simulink model "attempt_at_model"  (R2024a)
settings: Solver=FixedStepAuto  StartTime=0.0  StopTime=inf  RelTol=1e-3
model workspace (MAT data in the model file):
  SL_ROS_VariableLengthArrays_MaxSizes.CommonInfo.ArrayTruncateAction = 'EmitWarning'
  SL_ROS_VariableLengthArrays_MaxSizes.MsgTypeMap = containers.Map
  SL_ROS_VariableLengthArrays_MaxSizes.MsgTypeMap.serialization.keys = {'sensor_msgs/CompressedImage'}
  SL_ROS_VariableLengthArrays_MaxSizes.MsgTypeMap.serialization.values{1}(1).PropertyName = 'data'
  SL_ROS_VariableLengthArrays_MaxSizes.MsgTypeMap.serialization.values{1}(1).DataType = 'uint8'
  SL_ROS_VariableLengthArrays_MaxSizes.MsgTypeMap.serialization.values{1}(1).MaxLength = 87917
  SL_ROS_VariableLengthArrays_MaxSizes.MsgTypeMap.serialization.values{1}(2).PropertyName = 'format'
  SL_ROS_VariableLengthArrays_MaxSizes.MsgTypeMap.serialization.values{1}(2).DataType = 'uint8'
  SL_ROS_VariableLengthArrays_MaxSizes.MsgTypeMap.serialization.values{1}(2).MaxLength = 128
  SL_ROS_VariableLengthArrays_MaxSizes.MsgTypeMap.serialization.uniformity = 0
  SL_ROS_VariableLengthArrays_MaxSizes.MsgTypeMap.serialization.keyType = 'char'
  SL_ROS_VariableLengthArrays_MaxSizes.MsgTypeMap.serialization.valueType = 'any'
undefined symbols (not defined in the file): angular, fractalcoef, linear, theta, x, y
libraries: ros2lib x19, instrumentlib x5, mspsensorlib x1, visionsinks x1
settings Model: Creator=RedBlueBerry177  LastModifiedBy=ejsui
settings OptimizationCC: EnhancedBackFolding=on  PassReuseOutputArgsAs=Individual arguments  ZeroExternalMemoryAtStartup=off  ZeroInternalMemoryAtStartup=off  MaxStackSize=64  OptimizeBlockOrder=speed  DifferentSizesBufferReuse=on  OptimizationCustomize=off  EfficientTunableParamExpr=on
settings DebuggingCC: ParameterTunabilityLossMsg=error
settings SFSimCC: MATLABDynamicMemAlloc=off  SimTargetLang=C++
settings RTWCC: Description=Embedded Coder  SystemTargetFile=ert.tlc  HardwareBoard=Robot Operating System 2 (ROS 2)  TLCOptions="-aInlineSetEventsForThisBaseRateFcn=TLC_FALSE -aSuppressMultiTaskScheduler=TLC_FALSE  -aRateBasedStepFcn=0"  TemplateMakefile=ert_default_tmf  Toolchain=Colcon Tools  TargetLang=C++  GPUComputeCapability=3.5
settings CodeAppCC: ForceParamTrailComments=on  IgnoreCustomStorageClasses=off  OperatorAnnotations=on  SimulinkDataObjDesc=on  SFDataObjDesc=on  InsertBlockDesc=on
settings ERTTargetCC: CodeInterfacePackaging=C++ class  RootIOFormat=Structure reference

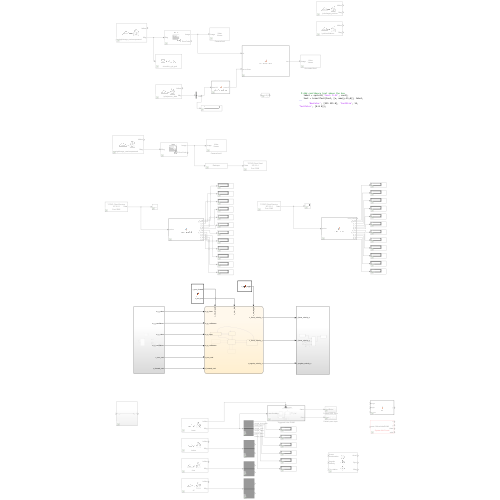
[thumbnail: Simulink's stored preview of the top-level diagram]
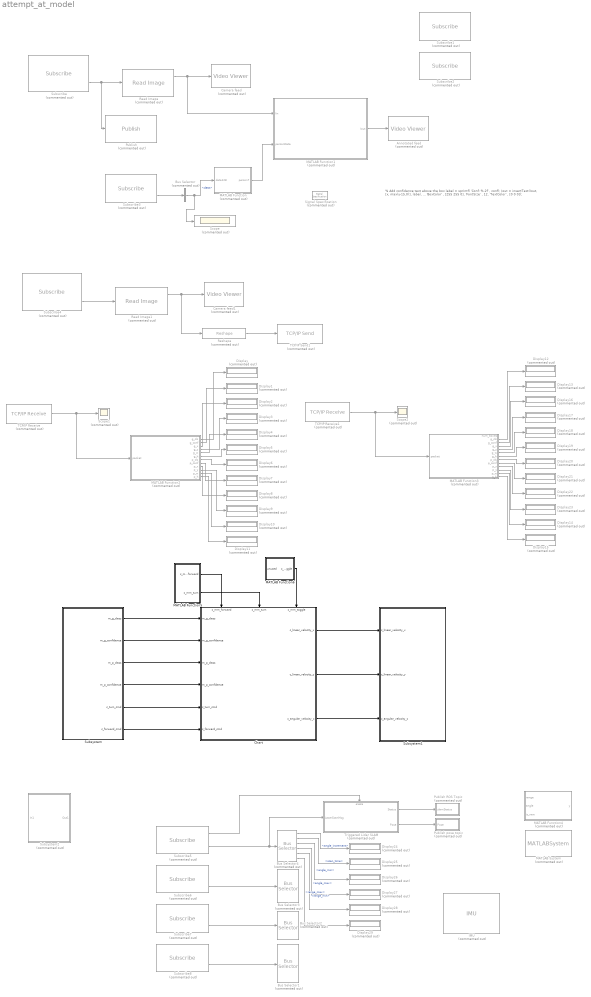
== system attempt_at_model ==
  note: % Add confidence text above the box
      | label = sprintf( 'Conf: %.2f' , conf);
      | Iout = insertText(Iout, [x, max(y-15,0)], label, ...
      | 'BoxColor' , [255 255 0], 'FontSize' , 12, 'TextColor' , [0 0 0]);
  Annotated feed : VideoViewer  Commented=on  FigPos=[1005 760 624 399]
  Bus Selector : BusSelector  Commented=on  OutputSignals=data
  Bus Selector1 : BusSelector  Commented=on  OutputSignals=signal1,signal2
  Bus Selector2 : BusSelector  Commented=on  OutputSignals=signal1,signal2
  Bus Selector3 : BusSelector  Commented=on  OutputSignals=signal1,signal2
  Bus Selector4 : BusSelector  Commented=on  OutputSignals=angle_increment,scan_time,angle_min,angle_max,range_min,range_max
  Camera feed : VideoViewer  Commented=on  FigPos=[409 769 608 539]
  Camera feed1 : VideoViewer  Commented=on  FigPos=[409 769 608 539]
  Chart : Stateflow chart  TreatAsAtomicUnit=on
      settings: PortSchema="{\"entries\":[{\"content\":{\"sides\":[{\"content\":{\"connectorIds\":[\"In4\",\"In5\",\"In6\",\"In7\",\"In8\",\"In9\"]},\"type\":\"ConnectorPlacement.EquallySpacedRectSide\",\"uuid\":\"6869af31-0483-4a0d-a5aa-348304382b03\"},{\"content\":{\"connectorIds\":[\"Out1\",\"Out2\",\"Out3\"],\"side\":\"RIGHT\"},\"type\":\"ConnectorPlacement.EquallySpacedRectSide\",\"uuid\":\"19448461-0885-46d3-901b-79cbd3d2f2eb\"},{\"content\":{\"connectorIds\":[\"In1\",\"In2\",\"In3\"],\"side\":\"TOP\"},\"type\":\"ConnectorPlacement.EquallySpacedRectSide\",\"uuid\":\"dcdfc426-3300-4bb7-b0c9-b15241839ab0\"}]},\"type\":\"ConnectorPlacement.EquallySpacedConnector\",\"uuid\":\"e0f68e20-794f-48c9-96e4-1765267eb054\"}],\"packageUris\":[\"http://schema.mathworks.com/mf0/Connector/R2020b\"],\"version\":\"1.0\"}"
  Display{,1..29} (30 alike) : Display  Commented=on
  IMU : mspsensorlib/IMU  Commented=on  DispRefFrame=NED  TemperaturePort=off  Temperature=25  MagneticFieldPort=off  MagneticFieldNED=[ 27.5550, -2.4169, -16.0849 ]  MagneticFieldENU=[ -2.4169, 27.5550, 16.0849 ]  SeedDouble=67  SimulateUsing=Interpreted execution  AccelParamsMeasurementRange=Inf  AccelParamsResolution=0  AccelParamsConstantBias=[ 0, 0, 0 ]  AccelParamsAxesMisalignment=[ 100, 0, 0; 0, 100, 0; 0, 0, 100 ]  AccelParamsNoiseDensity=[ 0, 0, 0 ]  AccelParamsBiasInstability=[ 0, 0, 0 ]  AccelParamsBiasInstabilityNumerator=fractalcoef().Numerator  AccelParamsBiasInstabilityDenominator=fractalcoef().Denominator  AccelParamsRandomWalk=[ 0, 0, 0 ]  AccelParamsNoiseType=double-sided  AccelParamsTemperatureBias=[ 0, 0, 0 ]  AccelParamsTemperatureScaleFactor=[ 0, 0, 0 ]  GyroParamsMeasurementRange=Inf  GyroParamsResolution=0  GyroParamsConstantBias=[ 0, 0, 0 ]  GyroParamsAxesMisalignment=[ 100, 0, 0; 0, 100, 0; 0, 0, 100 ]  GyroParamsAccelerationBias=[ 0, 0, 0 ]  GyroParamsNoiseDensity=[ 0, 0, 0 ]  GyroParamsBiasInstability=[ 0, 0, 0 ]  GyroParamsBiasInstabilityNumerator=fractalcoef().Numerator  GyroParamsBiasInstabilityDenominator=fractalcoef().Denominator  GyroParamsRandomWalk=[ 0, 0, 0 ]  GyroParamsNoiseType=double-sided  GyroParamsTemperatureBias=[ 0, 0, 0 ]  GyroParamsTemperatureScaleFactor=[ 0, 0, 0 ]  MagParamsMeasurementRange=Inf  MagParamsResolution=0  MagParamsConstantBias=[ 0, 0, 0 ]  MagParamsAxesMisalignment=[ 100, 0, 0; 0, 100, 0; 0, 0, 100 ]  MagParamsNoiseDensity=[ 0, 0, 0 ]  MagParamsBiasInstability=[ 0, 0, 0 ]  MagParamsBiasInstabilityNumerator=fractalcoef().Numerator  MagParamsBiasInstabilityDenominator=fractalcoef().Denominator  MagParamsRandomWalk=[ 0, 0, 0 ]  MagParamsNoiseType=double-sided  MagParamsTemperatureBias=[ 0, 0, 0 ]  MagParamsTemperatureScaleFactor=[ 0, 0, 0 ]
  MATLAB Function : MATLAB Function  Commented=on  TreatAsAtomicUnit=on
  MATLAB Function1 : MATLAB Function  Commented=on  TreatAsAtomicUnit=on
  MATLAB Function2 : MATLAB Function  Commented=on  TreatAsAtomicUnit=on
  MATLAB Function3 : MATLAB Function  Commented=on  TreatAsAtomicUnit=on
  MATLAB Function4 : MATLAB Function  Commented=on  TreatAsAtomicUnit=on
  MATLAB Function5 : MATLAB Function  TreatAsAtomicUnit=on
  MATLAB Function6 : MATLAB Function  TreatAsAtomicUnit=on
  MATLAB System : MATLABSystem  Commented=on  System=OnlineLidarSLAM  MapResolution=10  MaxRange=8.0  SimulateUsing=Code generation
      mask Type: OnlineLidarSLAM
      mask Display:
      | disp('OnlineLidarSLAM');
      | port_label('input',1,'scan');
      | port_label('output',1,'x');
      | port_label('output',2,'y');
      | port_label('output',3,'theta');
      | port_label('output',4,'valid');
  Publish : ros2lib/Publish  Commented=on  topicSource=Specify your own  topic=/simulink_rgb_pub  messageType=sensor_msgs/CompressedImage  QOSHistory=Keep last  QOSDepth=1  QOSReliability=Reliable  QOSDurability=Volatile  QOSDeadline=Inf  QOSLifespan=Inf  QOSLiveliness=Automatic  QOSLeaseDuration=Inf  QOSAvoidROSNamespaceConventions=off
  Publish ROS Topic : Subsystem  Commented=on
  Publish pose topic : Subsystem  Commented=on
  Read Image : ros2lib/Read Image  Commented=on  MaximumImageSize=[480,640]  ImageEncoding=rgb8  ShowAlphaOutput=off  ShowErrorCodeOutput=on  VariableSizeOutputs=off
  Read Image1 : ros2lib/Read Image  Commented=on  MaximumImageSize=[480,640]  ImageEncoding=rgb8  ShowAlphaOutput=off  ShowErrorCodeOutput=on  VariableSizeOutputs=off
  Reshape : Reshape  Commented=on  OutputDimensionality=Customize  OutputDimensions=[480 640 3]
  Scope : Scope  Commented=on
  Scope1 : Scope  Commented=on
  Scope2 : Scope  Commented=on
  Signal Specification : SignalSpecification  Commented=on  OutDataTypeStr=single  Dimensions=[1 7]
  Subscribe : ros2lib/Subscribe  Commented=on  topicSource=Select from ROS network  topic=/depth_cam/rgb/image_raw/compressed  messageType=sensor_msgs/CompressedImage  sampleTime=-1  QOSHistory=Keep last  QOSDepth=1  QOSReliability=Best effort  QOSDurability=Volatile  QOSDeadline=Inf  QOSLifespan=Inf  QOSLiveliness=Automatic  QOSLeaseDuration=Inf  QOSAvoidROSNamespaceConventions=off
  Subscribe1 : ros2lib/Subscribe  Commented=on  topicSource=Select from ROS network  topic=/yolo/target_position  messageType=geometry_msgs/Point  sampleTime=-1  QOSHistory=Keep last  QOSDepth=1  QOSReliability=Reliable  QOSDurability=Volatile  QOSDeadline=Inf  QOSLifespan=Inf  QOSLiveliness=Automatic  QOSLeaseDuration=Inf  QOSAvoidROSNamespaceConventions=off
  Subscribe2 : ros2lib/Subscribe  Commented=on  topicSource=Select from ROS network  topic=/yolo/confidence  messageType=std_msgs/Float32  sampleTime=-1  QOSHistory=Keep last  QOSDepth=1  QOSReliability=Reliable  QOSDurability=Volatile  QOSDeadline=Inf  QOSLifespan=Inf  QOSLiveliness=Automatic  QOSLeaseDuration=Inf  QOSAvoidROSNamespaceConventions=off
  Subscribe3 : ros2lib/Subscribe  Commented=on  topicSource=Select from ROS network  topic=/yolo/person_data  messageType=std_msgs/Float32MultiArray  sampleTime=-1  QOSHistory=Keep last  QOSDepth=1  QOSReliability=Reliable  QOSDurability=Volatile  QOSDeadline=Inf  QOSLifespan=Inf  QOSLiveliness=Automatic  QOSLeaseDuration=Inf  QOSAvoidROSNamespaceConventions=off
  Subscribe4 : ros2lib/Subscribe  Commented=on  topicSource=Select from ROS network  topic=/depth_cam/rgb/image_raw/compressed  messageType=sensor_msgs/CompressedImage  sampleTime=-1  QOSHistory=Keep last  QOSDepth=1  QOSReliability=Best effort  QOSDurability=Volatile  QOSDeadline=Inf  QOSLifespan=Inf  QOSLiveliness=Automatic  QOSLeaseDuration=Inf  QOSAvoidROSNamespaceConventions=off
  Subscribe5 : ros2lib/Subscribe  Commented=on  topicSource=Select from ROS network  topic=/scan  messageType=sensor_msgs/LaserScan  sampleTime=-1  QOSHistory=Keep last  QOSDepth=1  QOSReliability=Reliable  QOSDurability=Volatile  QOSDeadline=Inf  QOSLifespan=Inf  QOSLiveliness=Automatic  QOSLeaseDuration=Inf  QOSAvoidROSNamespaceConventions=off
  Subscribe6 : ros2lib/Subscribe  Commented=on  topicSource=Select from ROS network  topic=/odom  messageType=nav_msgs/Odometry  sampleTime=-1  QOSHistory=Keep last  QOSDepth=1  QOSReliability=Reliable  QOSDurability=Volatile  QOSDeadline=Inf  QOSLifespan=Inf  QOSLiveliness=Automatic  QOSLeaseDuration=Inf  QOSAvoidROSNamespaceConventions=off
  Subscribe7 : ros2lib/Subscribe  Commented=on  topicSource=Select from ROS network  topic=/imu  messageType=sensor_msgs/Imu  sampleTime=-1  QOSHistory=Keep last  QOSDepth=1  QOSReliability=Reliable  QOSDurability=Volatile  QOSDeadline=Inf  QOSLifespan=Inf  QOSLiveliness=Automatic  QOSLeaseDuration=Inf  QOSAvoidROSNamespaceConventions=off
  Subscribe8 : ros2lib/Subscribe  Commented=on  topicSource=Select from ROS network  topic=/tf  messageType=tf2_msgs/TFMessage  sampleTime=-1  QOSHistory=Keep last  QOSDepth=1  QOSReliability=Reliable  QOSDurability=Volatile  QOSDeadline=Inf  QOSLifespan=Inf  QOSLiveliness=Automatic  QOSLeaseDuration=Inf  QOSAvoidROSNamespaceConventions=off
  Subsystem : Subsystem
  Subsystem1 : Subsystem
  Subsystem2 : Subsystem  Commented=on
  TCP/IP Receive : instrumentlib/TCP//IP Receive  Commented=on  Host=127.0.0.1  Port=5005  DataSize=[56, 1]  DataType=uint8  ASCIIFormatting=%f  Terminator=LF  CustomTerminator=10  ByteOrder=big-endian  EnableBlockingMode=on  Timeout=1000  SampleTime=0.01  SimulateUsing=Interpreted execution
  TCP/IP Receive1 : instrumentlib/TCP//IP Receive  Commented=on  Host=127.0.0.1  Port=5005  DataSize=[52, 1]  DataType=uint8  ASCIIFormatting=%f  Terminator=LF  CustomTerminator=10  ByteOrder=big-endian  EnableBlockingMode=on  Timeout=1000  SampleTime=0.01  SimulateUsing=Interpreted execution
  TCP/IP Send1 : instrumentlib/TCP//IP Send  Commented=on  Host=127.0.0.1  Port=5005  ByteOrder=big-endian  EnableBlockingMode=on  Timeout=10  TransferDelay=off  SimulateUsing=Interpreted execution
  Triggered Lidar SLAM : Subsystem  Commented=on
  wires:
  Subscribe/2 -> Publish/1, Read Image/1
  Read Image/1 -> MATLAB Function1/1(Iin), Camera feed/1
  MATLAB Function1/1(Iout) -> Annotated feed/1
  Subscribe3/2 -> Bus Selector/1
  Bus Selector/1 -> Scope/1, MATLAB Function/1(data128)  "<data>"
  MATLAB Function/1(person7) -> MATLAB Function1/2(personData)
  Subscribe4/2 -> Read Image1/1
  Read Image1/1 -> Reshape/1, Camera feed1/1
  Reshape/1 -> TCP/IP Send1/1
  TCP/IP Receive/1 -> MATLAB Function2/1(packet), Scope1/1
  MATLAB Function2/1(g_cls) -> Display/1
  MATLAB Function2/2(g_conf) -> Display1/1
  MATLAB Function2/3(g_x) -> Display2/1
  MATLAB Function2/4(g_y) -> Display3/1
  MATLAB Function2/5(g_w) -> Display4/1
  MATLAB Function2/6(g_h) -> Display5/1
  MATLAB Function2/7(p_cls) -> Display6/1
  MATLAB Function2/8(p_conf) -> Display7/1
  MATLAB Function2/9(p_x) -> Display8/1
  MATLAB Function2/10(p_y) -> Display9/1
  MATLAB Function2/11(p_w) -> Display10/1
  MATLAB Function2/12(p_h) -> Display11/1
  MATLAB Function3/8(p_cls) -> Display20/1
  MATLAB Function3/12(p_w) -> Display14/1
  MATLAB Function3/11(p_y) -> Display23/1
  MATLAB Function3/9(p_conf) -> Display21/1
  MATLAB Function3/10(p_x) -> Display22/1
  MATLAB Function3/2(g_cls) -> Display12/1
  MATLAB Function3/13(p_h) -> Display15/1
  MATLAB Function3/6(g_w) -> Display18/1
  MATLAB Function3/4(g_x) -> Display16/1
  MATLAB Function3/5(g_y) -> Display17/1
  TCP/IP Receive1/1 -> MATLAB Function3/1(packet), Scope2/1
  MATLAB Function3/3(g_conf) -> Display13/1
  MATLAB Function3/7(g_h) -> Display19/1
  Subsystem/1(m_g_class) -> Chart/4(m_g_class)
  Subsystem/2(m_g_confidence) -> Chart/5(m_g_confidence)
  Subsystem/3(m_p_class) -> Chart/6(m_p_class)
  Subsystem/4(m_p_confidence) -> Chart/7(m_p_confidence)
  Chart/1(c_linear_velocity_x) -> Subsystem1/1(c_linear_velocity_x)
  Chart/2(c_linear_velocity_y) -> Subsystem1/2(c_linear_velocity_y)
  Subsystem/5(c_turn_cmd) -> Chart/8(c_turn_cmd)
  Subsystem/6(c_forward_cmd) -> Chart/9(c_forward_cmd)
  Chart/3(c_angular_velocity_z) -> Subsystem1/3(c_angular_velocity_z)
  Subscribe8/2 -> Bus Selector1/1
  Subscribe7/2 -> Bus Selector2/1
  Subscribe6/2 -> Bus Selector3/1
  Subscribe5/2 -> Triggered Lidar SLAM/1(LaserScanMsg), Bus Selector4/1
  Subscribe5/1 -> Triggered Lidar SLAM/Enable
  Triggered Lidar SLAM/1(Status) -> Publish ROS Topic/1(slamStatus)
  Triggered Lidar SLAM/2(Pose) -> Publish pose topic/1(Pose)
  Bus Selector4/1 -> Display24/1  "<angle_increment>"
  Bus Selector4/2 -> Display25/1  "<scan_time>"
  Bus Selector4/3 -> Display26/1  "<angle_min>"
  Bus Selector4/4 -> Display27/1  "<angle_max>"
  Bus Selector4/5 -> Display28/1  "<range_min>"
  Bus Selector4/6 -> Display29/1  "<range_max>"
  MATLAB Function5/1(c_mm_forward) -> Chart/1(c_mm_forward)
  MATLAB Function5/2(c_mm_turn) -> Chart/2(c_mm_turn)
  MATLAB Function6/1(c_mm_toggle) -> Chart/3(c_mm_toggle)

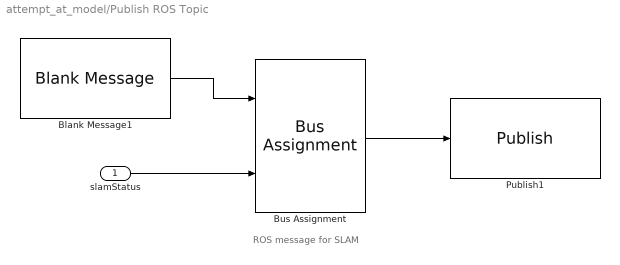
== system attempt_at_model/Publish ROS Topic ==
  note: ROS message for SLAM
  slamStatus : Inport
  Blank Message1 : ros2lib/Blank Message  messageClass=Message  entityType=std_msgs/Int8  messageType=std_msgs/Int8  SampleTime=inf
  Bus Assignment : BusAssignment  AssignedSignals=data
  Publish1 : ros2lib/Publish  topicSource=Specify your own  topic=/slamStatus  messageType=std_msgs/Int8  QOSHistory=Keep last  QOSDepth=1  QOSReliability=Reliable  QOSDurability=Volatile  QOSDeadline=Inf  QOSLifespan=Inf  QOSLiveliness=Automatic  QOSLeaseDuration=Inf  QOSAvoidROSNamespaceConventions=off
  wires:
  slamStatus/1 -> Bus Assignment/2
  Blank Message1/1 -> Bus Assignment/1
  Bus Assignment/1 -> Publish1/1

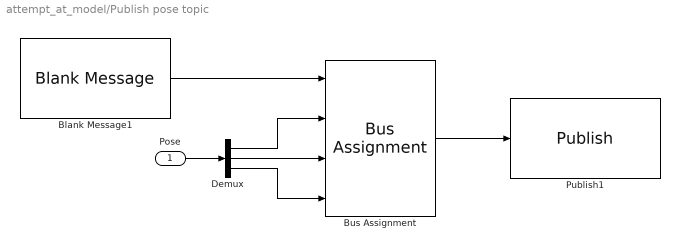
== system attempt_at_model/Publish pose topic ==
  Pose : Inport
  Blank Message1 : ros2lib/Blank Message  messageClass=Message  entityType=geometry_msgs/Pose2D  messageType=geometry_msgs/Pose2D  SampleTime=inf
  Bus Assignment : BusAssignment  AssignedSignals=x,y,theta
  Demux : Demux  Outputs=3
  Publish1 : ros2lib/Publish  topicSource=Specify your own  topic=/pose  messageType=geometry_msgs/Pose2D  QOSHistory=Keep last  QOSDepth=1  QOSReliability=Reliable  QOSDurability=Volatile  QOSDeadline=Inf  QOSLifespan=Inf  QOSLiveliness=Automatic  QOSLeaseDuration=Inf  QOSAvoidROSNamespaceConventions=off
  wires:
  Pose/1 -> Demux/1
  Demux/3 -> Bus Assignment/4
  Demux/1 -> Bus Assignment/2
  Demux/2 -> Bus Assignment/3
  Blank Message1/1 -> Bus Assignment/1
  Bus Assignment/1 -> Publish1/1

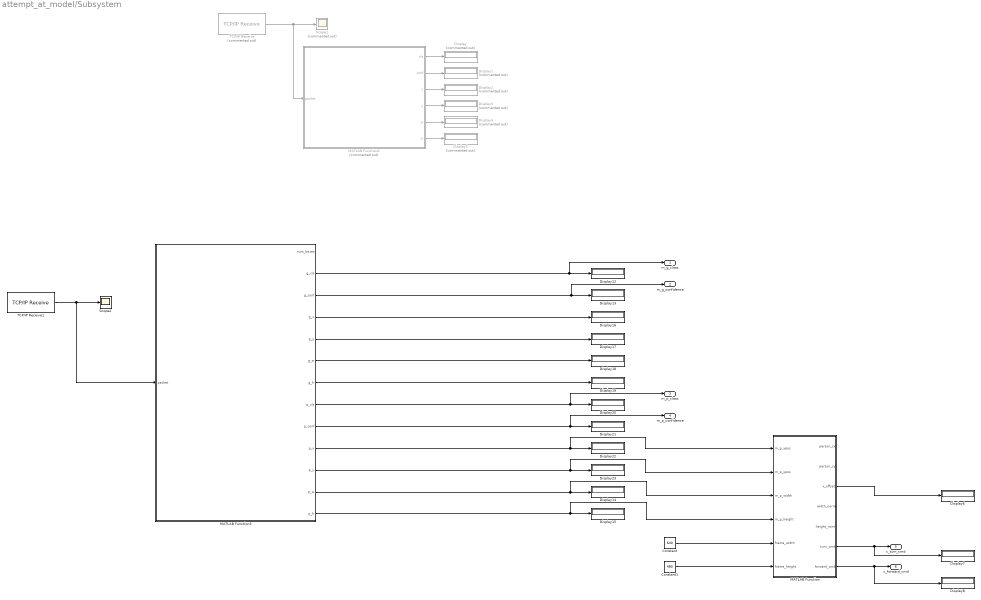
== system attempt_at_model/Subsystem ==
  Constant : Constant  Value=640
  Constant1 : Constant  Value=480
  Display{,1..5} (6 alike) : Display  Commented=on
  Display{6..8,12..23} (15 alike) : Display
  MATLAB Function : MATLAB Function  TreatAsAtomicUnit=on
  MATLAB Function2 : MATLAB Function  Commented=on  TreatAsAtomicUnit=on
  MATLAB Function3 : MATLAB Function  TreatAsAtomicUnit=on
  Scope1 : Scope  Commented=on
  Scope2 : Scope
  TCP/IP Receive : instrumentlib/TCP//IP Receive  Commented=on  Host=127.0.0.1  Port=5005  DataSize=[28, 1]  DataType=uint8  ASCIIFormatting=%f  Terminator=LF  CustomTerminator=10  ByteOrder=big-endian  EnableBlockingMode=on  Timeout=1000  SampleTime=0.01  SimulateUsing=Interpreted execution
  TCP/IP Receive1 : instrumentlib/TCP//IP Receive  Host=127.0.0.1  Port=5005  DataSize=[52, 1]  DataType=uint8  ASCIIFormatting=%f  Terminator=LF  CustomTerminator=10  ByteOrder=big-endian  EnableBlockingMode=on  Timeout=1000  SampleTime=0.01  SimulateUsing=Interpreted execution
  m_g_class : Outport
  m_g_confidence : Outport  Port=2
  m_p_class : Outport  Port=3
  m_p_confidence : Outport  Port=4
  c_turn_cmd : Outport  Port=5
  c_forward_cmd : Outport  Port=6
  wires:
  MATLAB Function2/1(cls) -> Display/1
  MATLAB Function2/4(y) -> Display3/1
  MATLAB Function2/6(h) -> Display5/1
  MATLAB Function2/3(x) -> Display2/1
  MATLAB Function2/5(w) -> Display4/1
  TCP/IP Receive/1 -> MATLAB Function2/1(packet), Scope1/1
  MATLAB Function2/2(conf) -> Display1/1
  MATLAB Function3/9(p_conf) -> m_p_confidence/1, Display21/1
  MATLAB Function3/6(g_w) -> Display18/1
  MATLAB Function3/4(g_x) -> Display16/1
  MATLAB Function3/13(p_h) -> MATLAB Function/4(m_p_height), Display15/1
  MATLAB Function3/10(p_x) -> MATLAB Function/1(m_p_xpos), Display22/1
  MATLAB Function3/7(g_h) -> Display19/1
  MATLAB Function3/8(p_cls) -> m_p_class/1, Display20/1
  MATLAB Function3/11(p_y) -> MATLAB Function/2(m_p_ypos), Display23/1
  MATLAB Function3/3(g_conf) -> m_g_confidence/1, Display13/1
  MATLAB Function3/2(g_cls) -> m_g_class/1, Display12/1
  MATLAB Function3/5(g_y) -> Display17/1
  TCP/IP Receive1/1 -> MATLAB Function3/1(packet), Scope2/1
  MATLAB Function3/12(p_w) -> MATLAB Function/3(m_p_width), Display14/1
  Constant/1 -> MATLAB Function/5(frame_width)
  Constant1/1 -> MATLAB Function/6(frame_height)
  MATLAB Function/3(x_offset) -> Display6/1
  MATLAB Function/6(turn_cmd) -> Display7/1, c_turn_cmd/1
  MATLAB Function/7(forward_cmd) -> Display8/1, c_forward_cmd/1

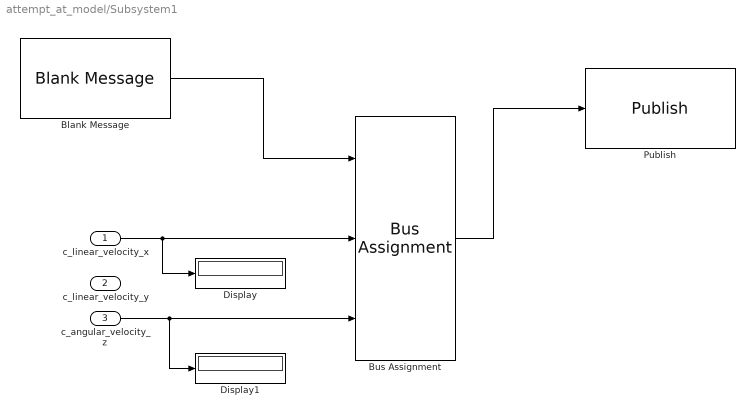
== system attempt_at_model/Subsystem1 ==
  c_linear_velocity_x : Inport
  c_linear_velocity_y : Inport  Port=2
  c_angular_velocity_z : Inport  Port=3
  Blank Message : ros2lib/Blank Message  messageClass=Message  entityType=geometry_msgs/Twist  messageType=geometry_msgs/Twist  SampleTime=inf
  Bus Assignment : BusAssignment  AssignedSignals=linear.x,angular.z
  Display : Display
  Display1 : Display
  Publish : ros2lib/Publish  topicSource=Select from ROS network  topic=/controller/cmd_vel  messageType=geometry_msgs/Twist  QOSHistory=Keep last  QOSDepth=1  QOSReliability=Reliable  QOSDurability=Volatile  QOSDeadline=Inf  QOSLifespan=Inf  QOSLiveliness=Automatic  QOSLeaseDuration=Inf  QOSAvoidROSNamespaceConventions=off
  wires:
  Blank Message/1 -> Bus Assignment/1
  c_linear_velocity_x/1 -> Display/1, Bus Assignment/2
  Bus Assignment/1 -> Publish/1
  c_angular_velocity_z/1 -> Display1/1, Bus Assignment/3

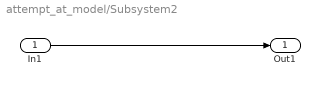
== system attempt_at_model/Subsystem2 ==
  In1 : Inport
  Out1 : Outport
  wires:
  In1/1 -> Out1/1

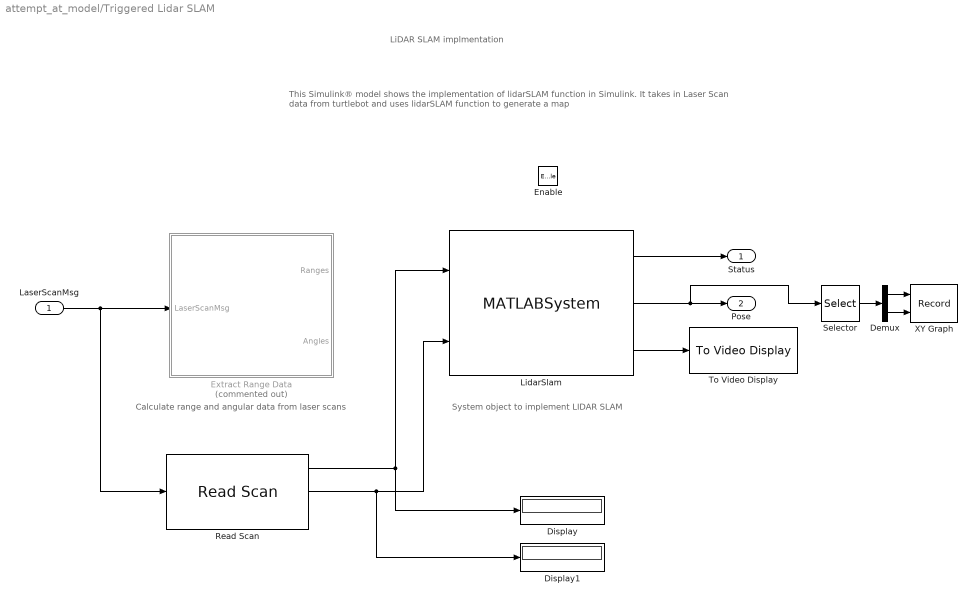
== system attempt_at_model/Triggered Lidar SLAM ==
  note: Calculate range and angular data from laser scans
  note: LiDAR SLAM implmentation
  note: This Simulink® model shows the implementation of lidarSLAM function in Simulink. It takes in Laser Scan data from turtlebot and uses lidarSLAM function to generate a map
  note: System object to implement LIDAR SLAM
  LaserScanMsg : Inport
  Enable : EnablePort  PropagateVarSize=During execution
  Demux : Demux  Outputs=2
  Display : Display
  Display1 : Display
  Extract Range Data : MATLAB Function  Commented=on  TreatAsAtomicUnit=on
  LidarSlam : MATLABSystem  System=LidarSlam_interp  SimulateUsing=Interpreted execution
      mask Type: LidarSlam_interp
      mask Display:
      | disp('LidarSlam_interp');
      | port_label('input',1,'ranges');
      | port_label('input',2,'angles');
      | port_label('output',1,'slamStatus');
      | port_label('output',2,'pose');
      | port_label('output',3,'mapData');
  Read Scan : ros2lib/Read Scan  MaximumArrayLength=1000  ShowAnglesOutput=on  ShowIntensityOutput=off  ShowErrorCodeOutput=on  VariableSizeOutputs=off
  Selector : Selector  InputPortWidth=3  IndexOptions=Index vector (dialog)  Indices=[1 2]  OutputSizes=1
  To Video Display : visionsinks/To Video Display  windowSizeMode=Normal  openAtMdlStart=on  fullScreen=off  videoWindowX=536805376  videoWindowY=536805376  saveWindowSize=off  videoWindowWidth=1000  videoWindowHeight=1000  inputColorFormat=RGB  inputType=Obsolete  imagePorts=One multidimensional signal  OutputDevice=On-screen video monitor  dataOrg=Column-major  isWindowOpen=off
  XY Graph : Record  FileSettingsInternal="{\"entries\":[{\"content\":{\"excelSettings\":{\"content\":{},\"type\":\"Streamout.ExcelSettings\"}},\"type\":\"Streamout.FileSettingStorage\",\"uuid\":\"\"}],\"packageUris\":[\"http:\\/\\/schema.mathworks.com\\/mf0\\/streamout_blocks\\/R2020a\"],\"version\":\"1.0\"}"  Layout=[1 1]  SignalsInternal="{\"entries\":[{\"content\":{\"signals\":[{\"content\":{\"blockPath\":[],\"dimensions\":[1,1],\"domain\":\"\",\"lineColor\":\"#a2142f\",\"plots\":[ 1 ],\"port\":1,\"signalID\":1,\"signalName\":\"Demux:1\"},\"type\":\"RecordBlkView.Signal\",\"uuid\":\"\"},{\"content\":{\"blockPath\":[],\"dimensions\":[1,1],\"domain\":\"\",\"lineColor\":\"#139fff\",\"plots\":[ 1 ],\"port\":2,\"signalID\":2,\"signalName\":\"Demux:2\"},\"type\":\"RecordBlkView.Signal\",\"uuid\":\"\"}]},\"type\":\"RecordBlkView.InputSignals\",\"uuid\":\"\"}],\"packageUris\":[\"http:\\/\\/schema.mathworks.com\\/mf0\\/streamout_blocks\\/R2020a\"],\"version\":\"1.0\"}"  VisualizationBindings="{\"xyplotplugin\":{\"info\":[{\"series\":[{\"bindingParametersList\":[{\"parameter\":\"X-Axis\",\"signalID\":1,\"signalName\":\"Demux:1\"},{\"parameter\":\"Y-Axis\",\"signalID\":2,\"signalName\":\"Demux:2\"}],\"seriesID\":0}],\"subplotID\":1}]}}"  CompatibilityTag=XY  st=-1
  Status : Outport
  Pose : Outport  Port=2
  wires:
  LaserScanMsg/1 -> Read Scan/1, Extract Range Data/1(LaserScanMsg)
  LidarSlam/1 -> Status/1
  LidarSlam/2 -> Pose/1, Selector/1
  Demux/2 -> XY Graph/2
  Demux/1 -> XY Graph/1
  Selector/1 -> Demux/1
  LidarSlam/3 -> To Video Display/1
  Read Scan/1 -> LidarSlam/1, Display/1
  Read Scan/2 -> Display1/1, LidarSlam/2

== stateflow chart attempt_at_model/Chart ==
  state Initial
  state Manual_Mode
    c_linear_velocity_x = c_mm_forward;
    c_angular_velocity_z = c_mm_turn;
  state Path_Planning_and_Navigation [commented out]
  state Idle
    c_linear_velocity_x = 0.0;
    c_linear_velocity_y = 0.0;
    c_angular_velocity_z = 0.0;
  state Follow
    c_linear_velocity_x = c_forward_cmd;
    c_linear_velocity_y = 0;
    c_angular_velocity_z = c_turn_cmd;
  state Mapping_and_Localization [commented out]
  Follow -> Manual_Mode [order 2] : [c_mm_toggle ==1]
  (default) -> Initial
  Initial -> Manual_Mode [order 2] : [c_mm_toggle == 1]
  Manual_Mode -> Initial : [c_mm_toggle == 0]
  Idle -> Manual_Mode [order 2] : [c_mm_toggle == 1]
  Initial -> Idle [order 1] : [(m_g_class == 9) & (m_p_class ==1)]
  Path_Planning_and_Navigation -> Idle [commented out]
  Idle -> Follow [order 1] : [m_g_class == 20]
  Idle -> Path_Planning_and_Navigation [commented out]
  Follow -> Idle [order 1] : [(m_g_class == 13) | (m_p_class == 0)]
  Idle -> Mapping_and_Localization [commented out] : [m_g_class == 13]
  Mapping_and_Localization -> Idle [commented out]
  data: c_mm_forward input; c_mm_turn input; c_mm_toggle input; m_g_class input; m_g_confidence input; m_p_class input; m_p_confidence input; c_linear_velocity_x output; c_linear_velocity_y output; c_turn_cmd input; c_forward_cmd input; c_angular_velocity_z output

== matlab function attempt_at_model/Subsystem/MATLAB Function2 ==
  data: packet input; cls output int32 size=1; conf output single size=1; x output single size=1; y output single size=1; w output single size=1; h output single size=1
function [cls, conf, x, y, w, h] = parse_packet(packet)
    cls  = typecast(packet(5:8), 'int32');       
    conf = typecast(packet(9:12), 'single');
    x    = typecast(packet(13:16), 'single');
    y    = typecast(packet(17:20), 'single');
    w    = typecast(packet(21:24), 'single');
    h    = typecast(packet(25:28), 'single');
end

== matlab function attempt_at_model/MATLAB Function3 ==
  data: num_boxes output uint32 size=1; packet input; g_cls output int32 size=1; g_conf output single size=1; g_x output single size=1; g_y output single size=1; g_w output single size=1; g_h output single size=1; p_cls output int32 size=1; p_conf output single size=1; p_x output single size=1; p_y output single size=1; p_w output single size=1; p_h output single size=1
function [num_boxes, g_cls, g_conf, g_x, g_y, g_w, g_h, p_cls, p_conf, p_x, p_y, p_w, p_h] = parse_packet(packet)

num_boxes = typecast(packet(1:4), 'uint32');

% Person box
p_cls  = typecast(packet(5:8), 'int32');
p_conf = typecast(packet(9:12), 'single');
p_x    = typecast(packet(13:16), 'single');
p_y    = typecast(packet(17:20), 'single');
p_w    = typecast(packet(21:24), 'single');
p_h    = typecast(packet(25:28), 'single');

% Gesture box
g_cls  = typecast(packet(29:32), 'int32');
g_conf = typecast(packet(33:36), 'single');
g_x    = typecast(packet(37:40), 'single');
g_y    = typecast(packet(41:44), 'single');
g_w    = typecast(packet(45:48), 'single');
g_h    = typecast(packet(49:52), 'single');
end

== matlab function attempt_at_model/Subsystem/MATLAB Function3 ==
  data: num_boxes output uint32 size=1; packet input; g_cls output int32 size=1; g_conf output single size=1; g_x output single size=1; g_y output single size=1; g_w output single size=1; g_h output single size=1; p_cls output int32 size=1; p_conf output single size=1; p_x output single size=1; p_y output single size=1; p_w output single size=1; p_h output single size=1
function [num_boxes, g_cls, g_conf, g_x, g_y, g_w, g_h, p_cls, p_conf, p_x, p_y, p_w, p_h] = parse_packet(packet)

num_boxes = typecast(packet(1:4), 'uint32');

% Person box
p_cls  = typecast(packet(5:8), 'int32');
p_conf = typecast(packet(9:12), 'single');
p_x    = typecast(packet(13:16), 'single');
p_y    = typecast(packet(17:20), 'single');
p_w    = typecast(packet(21:24), 'single');
p_h    = typecast(packet(25:28), 'single');

% Gesture box
g_cls  = typecast(packet(29:32), 'int32');
g_conf = typecast(packet(33:36), 'single');
g_x    = typecast(packet(37:40), 'single');
g_y    = typecast(packet(41:44), 'single');
g_w    = typecast(packet(45:48), 'single');
g_h    = typecast(packet(49:52), 'single');
end

== matlab function attempt_at_model/Subsystem/MATLAB Function ==
  data: m_p_xpos input; person_cx output; m_p_ypos input; m_p_width input; m_p_height input; frame_width input; frame_height input; person_cy output; x_offset output; width_norm output; height_norm output; turn_cmd output; forward_cmd output
function [person_cx, person_cy, x_offset, width_norm, height_norm, turn_cmd, forward_cmd] = compute_person_controls(m_p_xpos, m_p_ypos, m_p_width, m_p_height, frame_width, frame_height)
% Computes quantities for following a person in a frame
%
% Inputs:
%   m_p_xpos, m_p_ypos : top-left corner of person bounding box
%   m_p_width, m_p_height : width and height of bounding box
%   frame_width, frame_height : size of camera frame
%
% Outputs:
%   person_cx, person_cy : center of bounding box
%   x_offset : horizontal offset from frame center (pixels)
%   width_norm, height_norm : bounding box size normalized to frame size
%   turn_cmd : command for turning (-1=left, 0=centered, 1=right)
%   forward_cmd : command for forward movement (0=stop, 1=move)

% Compute center of bounding box
person_cx = m_p_xpos + m_p_width/2;
person_cy = m_p_ypos + m_p_height/2;

% Compute offset from frame center
x_offset = person_cx - frame_width/2;

% Normalize bounding box size
width_norm = m_p_width / frame_width;
height_norm = m_p_height / frame_height;

% ------------------------
% Turning logic
% ------------------------
x_threshold = 40; % pixels tolerance from center
if x_offset < -x_threshold
    turn_cmd = 0.2; % turn left
elseif x_offset > x_threshold
    turn_cmd = -0.2;  % turn right
else
    turn_cmd = 0;  % centered
end

% ------------------------
% Forward/backward logic
% ------------------------
desired_width = 0.8; % desired width of bounding box when at target distance
width_tolerance = 0.05;
if width_norm < (desired_width - width_tolerance)
    forward_cmd = 0.1; % move forward
else
    forward_cmd = 0; % stop
end

end

== matlab function attempt_at_model/MATLAB Function4 ==
  data: range input; y output; angle input; is_new input
function y = fcn(range, angle, is_new)
maxLidarRange = 8;
mapResolution = 20;
slamAlg = lidarSLAM(mapResolution, maxLidarRange, 100);
slamAlg.LoopClosureThreshold = 210;  
slamAlg.LoopClosureSearchRadius = 8;

if(is_new)
    scan = lidarScan(range,angle);
    [isScanAccepted, loopClosureInfo, optimizationInfo] = addScan(slamAlg, scan);
    if isScanAccepted
        fprintf('Added scan\n');
        figure;
        show(slamAlg);
    end
end

end

== matlab function attempt_at_model/Triggered Lidar SLAM/Extract Range Data ==
  data: LaserScanMsg input; Ranges output; Angles output
function [Ranges, Angles] = ExtractRangeData(LaserScanMsg)
%#codegen

% Extract Range information
Ranges = double(LaserScanMsg.Ranges);

% Construct Angles vector using AngleMin and AngleIncrement from sensor
% reading.
angMin = double(LaserScanMsg.AngleMin);
angIncrement = double(LaserScanMsg.AngleIncrement);

numReadings = numel(Ranges);
rawAngles = angMin + (0:numReadings-1)' * angIncrement;

% Wrap the angles to the (-pi,pi] interval.
Angles = robotics.internal.wrapToPi(double(rawAngles));

== matlab function attempt_at_model/MATLAB Function5 ==
  data: c_mm_forward output; c_mm_turn output
function [c_mm_forward, c_mm_turn] = fcn
%#codegen
% Initialize outputs
c_mm_forward = 0;
c_mm_turn = 0;


% Get key pressed in the current figure
k = get(gcf, 'CurrentCharacter');

if ~isempty(k)
    switch lower(k)
        case 'w'
            c_mm_forward = 0.1;
        case 'a'
            c_mm_turn = 0.2;
        case 's'
            c_mm_forward = -0.1;
        case 'd'
            c_mm_turn = -0.2;
    end
end

== matlab function attempt_at_model/MATLAB Function6 ==
  data: c_mm_toggle output; unused input
function c_mm_toggle = fcn(~)
%#codegen
% Toggle output each time 'm' is pressed

persistent toggle lastKey
if isempty(toggle)
    toggle = 0;      % current toggle state
    lastKey = '';    % previous key pressed
end

% Default output
c_mm_toggle = toggle;

% Get key pressed in the current figure
k = get(gcf, 'CurrentCharacter');

% Only toggle on a **new key press** (rising edge)
if ~isempty(k) && lower(k) == 'm' && ~strcmp(k, lastKey)
    toggle = ~toggle;  % flip state
    c_mm_toggle = toggle;
end

% Save last key pressed
if ~isempty(k)
    lastKey = k;
else
    lastKey = '';
end

== matlab function attempt_at_model/MATLAB Function1 ==
  data: Iin input; Iout output uint8 size=[480 640 3]; personData input single size=[1 7]
function Iout = drawPersonBox(Iin, personData)
% Iin         : Input RGB image (HxWx3)
% personData  : 1x7 Float32 array [x y w h cx cy confidence]

Iout = Iin;  % start with the original image

% Extract data
x = personData(1);
y = personData(2);
w = personData(3);
h = personData(4);
cx = personData(5);
cy = personData(6);
conf = personData(7);

% Only draw if confidence > 0
if conf > 0
    % Draw rectangle around detected person
    Iout = insertShape(Iout, 'Rectangle', [x, y, w, h], ...
        'Color', [0 255 0], 'LineWidth', 3);

  


end

== matlab function attempt_at_model/MATLAB Function ==
  data: data128 input; person7 output
function person7 = slicePersonData(data128)
% data128: [128x1] or [1x128]
person7 = reshape(data128(1:7), 1, 7);
end

== matlab function attempt_at_model/MATLAB Function2 ==
  data: packet input; g_cls output int32 size=1; g_conf output single size=1; g_x output single size=1; g_y output single size=1; g_w output single size=1; g_h output single size=1; p_cls output int32 size=1; p_conf output single size=1; p_x output single size=1; p_y output single size=1; p_w output single size=1; p_h output single size=1
function [g_cls, g_conf, g_x, g_y, g_w, g_h, ...
          p_cls, p_conf, p_x, p_y, p_w, p_h] = parse_packet(packet)

% ---------- Gesture ----------
g_cls  = typecast(packet(5:8),  'int32');
g_conf = typecast(packet(9:12), 'single');
g_x    = typecast(packet(13:16),'single');
g_y    = typecast(packet(17:20),'single');
g_w    = typecast(packet(21:24),'single');
g_h    = typecast(packet(25:28),'single');

% ---------- Person ----------
p_cls  = typecast(packet(33:36), 'int32');
p_conf = typecast(packet(37:40), 'single');
p_x    = typecast(packet(41:44), 'single');
p_y    = typecast(packet(45:48), 'single');
p_w    = typecast(packet(49:52), 'single');
p_h    = typecast(packet(53:56), 'single');

end
